simulink model "Sr12_threephase_pll_dq"  (Simulink 9.1)
settings: Solver=ode23s  StartTime=0.0  StopTime=0.2  MaxStep=1e-4  MinStep=1e-5  RelTol=1e-3  EnableMultiTasking=on
settings Model: Creator=suren  LastModifiedBy=Rajesh9
settings DataIOCC: LimitDataPoints=on  SignalLoggingSaveFormat=ModelDataLogs
settings OptimizationCC: ExpressionDepthLimit=2147483647  InitFltsAndDblsToZero=on
settings DebuggingCC: SaveWithParameterizedLinksMsg=none  SignalResolutionControl=TryResolveAllWithWarning  MultiTaskDSMMsg=warning  MultiTaskCondExecSysMsg=none  FcnCallInpInsideContextMsg=warning  StateNameClashWarn=warning
settings HardwareCC: TargetUnknown=on
settings GRTTargetCC: TargetFcnLib=ansi_tfl_tmw.mat  GeneratePreprocessorConditionals=Disable all

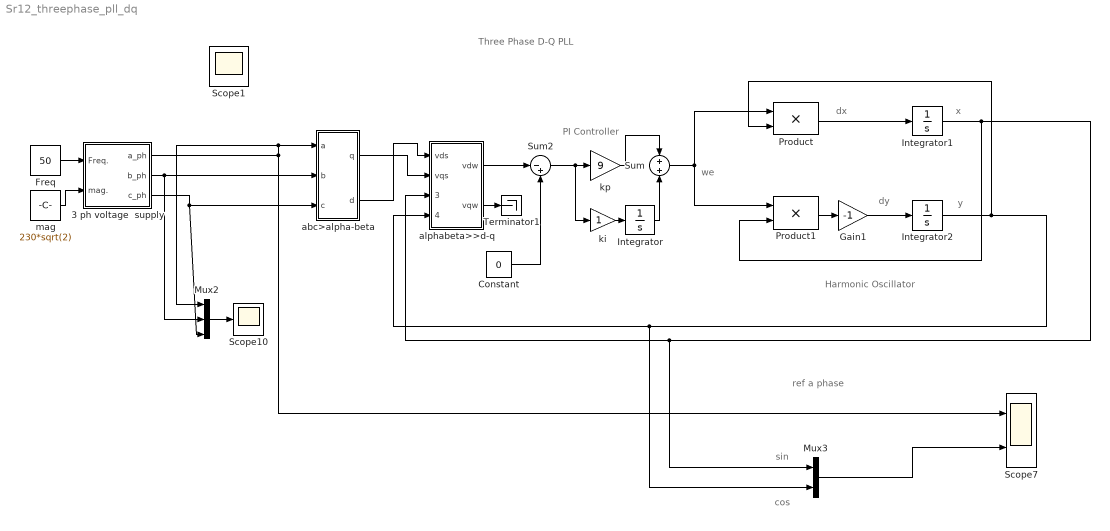
== system Sr12_threephase_pll_dq ==
  note: Three Phase D-Q PLL
  note: x
  note: y
  note: dx
  note: dy
  note: we
  note: sin
  note: cos
  note: ref a phase
  note: PI Controller
  note: Harmonic Oscillator
  3 ph voltage  supply : Subsystem
  Constant : Constant  Value=0  VectorParams1D=off
  Freq : Constant  Value=50
  Gain1 : Gain  Gain=-1  SaturateOnIntegerOverflow=on  OutDataTypeStr=Inherit: Same as input  ParamDataTypeStr=Inherit: Same as input
  Integrator : Integrator
  Integrator1 : Integrator  InitialCondition=1  LimitOutput=on  UpperSaturationLimit=1  LowerSaturationLimit=-1
  Integrator2 : Integrator  LimitOutput=on  UpperSaturationLimit=1  LowerSaturationLimit=-1
  Mux2 : Mux  Inputs=3
  Mux3 : Mux  Inputs=2
  Product : Product  SaturateOnIntegerOverflow=on  OutDataTypeStr=Inherit: Same as first input
  Product1 : Product  SaturateOnIntegerOverflow=on  OutDataTypeStr=Inherit: Same as first input
  Scope10 : Scope
  Scope7 : Scope  NumInputPorts=2
  Sum : Sum  SaturateOnIntegerOverflow=on
  Sum2 : Sum  Inputs=|-+  SaturateOnIntegerOverflow=on
  Terminator1 : Terminator
  abc>alpha-beta : Subsystem
  alphabeta>>d-q : Subsystem
  ki : Gain  SaturateOnIntegerOverflow=on  OutDataTypeStr=Inherit: Same as input  ParamDataTypeStr=Inherit: Same as input
  kp : Gain  Gain=9  SaturateOnIntegerOverflow=on  OutDataTypeStr=Inherit: Same as input  ParamDataTypeStr=Inherit: Same as input
  "mag " : Constant  Value=230*sqrt(2)
  Scope1 : Scope
  wires:
  Integrator2/1 -> Product/2, Mux3/2, alphabeta>>d-q/4(cos_e)
  Integrator1/1 -> Product1/2, Mux3/1, alphabeta>>d-q/3(sin_e)
  Product1/1 -> Gain1/1
  Product/1 -> Integrator1/1
  Freq/1 -> 3 ph voltage  supply/1(Freq.)
  "mag "/1 -> 3 ph voltage  supply/2(mag.)
  3 ph voltage  supply/1(a_ph) -> abc>alpha-beta/1(a), Mux2/1, Scope7/1
  3 ph voltage  supply/2(b_ph) -> abc>alpha-beta/2(b), Mux2/2
  3 ph voltage  supply/3(c_ph) -> abc>alpha-beta/3(c), Mux2/3
  abc>alpha-beta/1(q) -> alphabeta>>d-q/2(vqs)
  abc>alpha-beta/2(d) -> alphabeta>>d-q/1(vds)
  Gain1/1 -> Integrator2/1
  ki/1 -> Integrator/1
  Sum2/1 -> kp/1, ki/1
  kp/1 -> Sum/1
  Integrator/1 -> Sum/2
  Mux3/1 -> Scope7/2
  Mux2/1 -> Scope10/1
  Sum/1 -> Product1/1, Product/1
  alphabeta>>d-q/1(vdw) -> Sum2/1
  Constant/1 -> Sum2/2
  alphabeta>>d-q/2(vqw) -> Terminator1/1

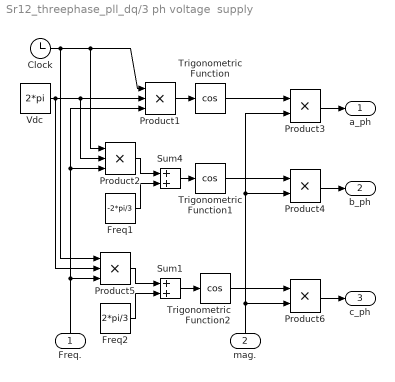
== system Sr12_threephase_pll_dq/3 ph voltage  supply ==
  Freq. : Inport
  mag. : Inport  Port=2
  Clock : Clock
  Freq1 : Constant  Value=-2*pi/3
  Freq2 : Constant  Value=2*pi/3
  Product1 : Product  Inputs=3  RndMeth=Zero
  Product2 : Product  Inputs=3  RndMeth=Zero
  Product3 : Product  RndMeth=Zero
  Product4 : Product  RndMeth=Zero
  Product5 : Product  Inputs=3  RndMeth=Zero
  Product6 : Product  RndMeth=Zero
  Sum1 : Sum  SaturateOnIntegerOverflow=on  InputSameDT=on  OutDataTypeStr=Inherit: Same as first input
  Sum4 : Sum  SaturateOnIntegerOverflow=on  InputSameDT=on  OutDataTypeStr=Inherit: Same as first input
  Trigonometric Function : Trigonometry  Operator=cos
  Trigonometric Function1 : Trigonometry  Operator=cos
  Trigonometric Function2 : Trigonometry  Operator=cos
  Vdc : Constant  Value=2*pi
  a_ph : Outport
  b_ph : Outport  Port=2
  c_ph : Outport  Port=3
  wires:
  Product1/1 -> Trigonometric Function/1
  Vdc/1 -> Product1/2, Product2/2, Product5/2
  Clock/1 -> Product1/1, Product2/1, Product5/1
  Freq./1 -> Product5/3, Product2/3, Product1/3
  Sum4/1 -> Trigonometric Function1/1
  Product2/1 -> Sum4/1
  Freq1/1 -> Sum4/2
  Trigonometric Function1/1 -> Product4/1
  Trigonometric Function/1 -> Product3/1
  Sum1/1 -> Trigonometric Function2/1
  Product5/1 -> Sum1/1
  Freq2/1 -> Sum1/2
  Trigonometric Function2/1 -> Product6/1
  mag./1 -> Product6/2, Product4/2, Product3/2
  Product3/1 -> a_ph/1
  Product4/1 -> b_ph/1
  Product6/1 -> c_ph/1

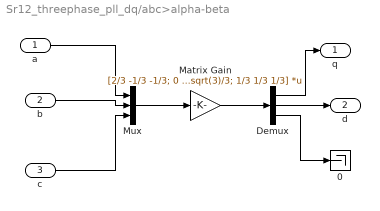
== system Sr12_threephase_pll_dq/abc>alpha-beta ==
  a : Inport
  b : Inport  Port=2
  c : Inport  Port=3
  0 : Terminator
  Demux : Demux  Outputs=3
  Matrix Gain : Gain  Gain=[2/3 -1/3 -1/3; 0 -sqrt(3)/3 sqrt(3)/3; 1/3 1/3 1/3]  Multiplication=Matrix(K*u)  SaturateOnIntegerOverflow=on  OutDataTypeStr=Inherit: Same as input  ParamDataTypeStr=Inherit: Same as input
  Mux : Mux  Inputs=3
  q : Outport
  d : Outport  Port=2
  wires:
  a/1 -> Mux/1
  b/1 -> Mux/2
  c/1 -> Mux/3
  Demux/1 -> q/1
  Demux/2 -> d/1
  Mux/1 -> Matrix Gain/1
  Matrix Gain/1 -> Demux/1
  Demux/3 -> 0/1

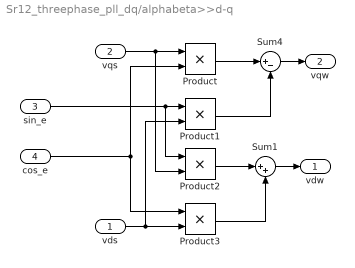
== system Sr12_threephase_pll_dq/alphabeta>>d-q ==
  vds : Inport
  vqs : Inport  Port=2
  sin_e : Inport  Port=3
  cos_e : Inport  Port=4
  Product{,1..3} (4 alike) : Product  SaturateOnIntegerOverflow=on  RndMeth=Zero  InputSameDT=on  OutDataTypeStr=Inherit: Same as first input
  Sum1 : Sum  Inputs=|++  SaturateOnIntegerOverflow=on  InputSameDT=on  OutDataTypeStr=Inherit: Same as first input
  Sum4 : Sum  Inputs=|+-  SaturateOnIntegerOverflow=on  InputSameDT=on  OutDataTypeStr=Inherit: Same as first input
  vdw : Outport
  vqw : Outport  Port=2
  wires:
  sin_e/1 -> Product1/1, Product2/1
  cos_e/1 -> Product/2, Product3/1
  vqs/1 -> Product2/2, Product/1
  vds/1 -> Product3/2, Product1/2
  Product/1 -> Sum4/1
  Product1/1 -> Sum4/2
  Product2/1 -> Sum1/1
  Product3/1 -> Sum1/2
  Sum4/1 -> vqw/1
  Sum1/1 -> vdw/1
